simulink model "cx06_MA"  (Simulink 7.5)
settings: Solver=FixedStepDiscrete  StartTime=0.0  StopTime=10.0  RelTol=1e-3
undefined symbols (not defined in the file or in its folder): DiscIntNeverNeededParam, ECU555, int, motohawk_build_version, motohawk_trunc_name, motohawk_vardec_path
libraries: MotoHawk_lib x811, simulink x43, simulink_need_slupdate x1
(part 10 of 10)

== system cx06_MA/Strategy/Hybrid Control Code/Regen/SOC_RampOut ==
  Torque_In : Inport  OutDataType=sfix(16)  OutScaling=2^0
  SOC : Inport  Port=2  OutDataType=sfix(16)  OutScaling=2^0
  Constant : Constant  OutDataType=sfix(16)  OutScaling=2^0
  Divide : Product  Inputs=*/  OutDataType=sfix(16)  OutScaling=2^-10
  Product : Product  OutDataType=sfix(16)  OutScaling=2^0  RndMeth=Zero
  Relational Operator : RelationalOperator  Operator=<=  LogicOutDataTypeMode=boolean  OutDataTypeStr=boolean
  Saturation : Saturate  UpperLimit=1  LowerLimit=0
  Sum : Sum  Inputs=-++  OutDataType=sfix(16)  OutScaling=2^0
  Switch : Switch  Criteria=u2 ~= 0
  motohawk_calibration : MotoHawk_lib/Calibration & Probing Blocks/motohawk_calibration  nam='RegenSOCRampWidth'  val=5  storage=Calibration  show_more=on  name_source=Use Parameter  data_type=Inherit from 'Default Value'  read_level=1  write_level=1  ovr_cals=on  view_as=Number  enum_struct={'Disabled', 'Enabled'}  vector_style=Wide Row  use_help_units=on  help='Regen ramps out this fast over max SOC'  units='%'  use_header_enum=off  row_header_enum={}  col_header_enum={}  use_min_max=on  min_val=0  max_val=100  use_precision=off  precision=''  gain=1  offset=0  exp=1  use_mototune_group=off  mototune_group=motohawk_vardec_path(gcb)
  motohawk_calibration1 : MotoHawk_lib/Calibration & Probing Blocks/motohawk_calibration  nam='RegenMaxSOC'  val=90  storage=Calibration  show_more=on  name_source=Use Parameter  data_type=Inherit from 'Default Value'  read_level=1  write_level=1  ovr_cals=on  view_as=Number  enum_struct={'Disabled', 'Enabled'}  vector_style=Wide Row  use_help_units=on  help='Max SOC to Regen At'  units='%'  use_header_enum=off  row_header_enum={}  col_header_enum={}  use_min_max=on  min_val=0  max_val=100  use_precision=off  precision=''  gain=1  offset=0  exp=1  use_mototune_group=off  mototune_group=motohawk_vardec_path(gcb)
  Torque_Out : Outport  OutDataType=sfix(16)  OutScaling=2^0
  wires:
  Product/1 -> Torque_Out/1
  Switch/1 -> Saturation/1
  Torque_In/1 -> Product/1
  Constant/1 -> Switch/1
  Divide/1 -> Switch/3
  Relational Operator/1 -> Switch/2
  motohawk_calibration/1 -> Divide/2, Sum/3
  Sum/1 -> Divide/1
  SOC/1 -> Sum/1, Relational Operator/1
  motohawk_calibration1/1 -> Sum/2, Relational Operator/2
  Saturation/1 -> Product/2

== system cx06_MA/Strategy/Hybrid Control Code/Regen/speed_RampOut ==
  note: Include a sign reversal for reverse regen here.
      | This will keep a consistant pedal feel.
  Torque_In : Inport  OutDataType=sfix(16)  OutScaling=2^0
  speed : Inport  Port=2  OutDataType=sfix(16)  OutScaling=2^0
  Abs : Abs
  Constant : Constant  OutDataType=sfix(16)  OutScaling=2^0
  Divide : Product  Inputs=*/  OutDataType=sfix(16)  OutScaling=2^-10
  Product : Product  Inputs=3  OutDataType=sfix(16)  OutScaling=2^0  RndMeth=Zero
  Relational Operator : RelationalOperator  Operator=>  LogicOutDataTypeMode=boolean  OutDataTypeStr=boolean
  Saturation : Saturate  UpperLimit=1  LowerLimit=0
  Sign : Signum
  Sum : Sum  Inputs=+-  OutDataType=sfix(16)  OutScaling=2^0
  Sum1 : Sum  Inputs=-+  OutDataType=sfix(16)  OutScaling=2^0
  Switch : Switch  Criteria=u2 ~= 0
  motohawk_data_def : MotoHawk_lib/Data Storage Blocks/motohawk_data_def  nam='RegenSpdRampStop'  container_nam=''  data=2  typ=double  struct_nam='MyStruct'  storage=NonVolatile  outputRef=off  use_vardec=on  window=Calibration  read_level=1  write_level=1  ovr_cals=on  view_as=Number  enum_struct={'Disabled', 'Enabled'}  vector_style=Wide Row  use_help_units=on  help='Speed at which regen is ramped out'  units='mph'  use_header_enum=off  row_header_enum=''  col_header_enum=''  use_min_max=on  min_val=0  max_val=100  use_precision=on  precision=''  gain=1  offset=0  exp=1  use_mototune_group=off  mototune_group=motohawk_vardec_path(gcb)  eval_name=RegenSpdRampStop  data_stores=motohawk_sfun_data_def_data_stores  struct_instances=motohawk_sfun_data_def_struct_instances  vardecs=motohawk_sfun_data_def_vardecs
  motohawk_data_def1 : MotoHawk_lib/Data Storage Blocks/motohawk_data_def  nam='RegenSpdRampStart'  container_nam=''  data=5  typ=double  struct_nam='MyStruct'  storage=NonVolatile  outputRef=off  use_vardec=on  window=Calibration  read_level=1  write_level=1  ovr_cals=on  view_as=Number  enum_struct={'Disabled', 'Enabled'}  vector_style=Wide Row  use_help_units=on  help='Speed at which regen starts to ramp out'  units='mph'  use_header_enum=off  row_header_enum=''  col_header_enum=''  use_min_max=off  min_val=0  max_val=100  use_precision=off  precision=''  gain=1  offset=0  exp=1  use_mototune_group=off  mototune_group=motohawk_vardec_path(gcb)  eval_name=RegenSpdRampStart  data_stores=motohawk_sfun_data_def_data_stores  struct_instances=motohawk_sfun_data_def_struct_instances  vardecs=motohawk_sfun_data_def_vardecs
  motohawk_data_read : MotoHawk_lib/Data Storage Blocks/motohawk_data_read  source=Lookup By Name  structure=Scalar  operation=Read scalar from location by index  sz_vec=4  sz_row=2  sz_col=3  typ=double  nam='RegenSpdRampStop'  checkNull=on  struct_inst_name='Struct1'  struct_nam='MyStruct'
  motohawk_data_read1 : MotoHawk_lib/Data Storage Blocks/motohawk_data_read  source=Lookup By Name  structure=Scalar  operation=Read scalar from location by index  sz_vec=4  sz_row=2  sz_col=3  typ=double  nam='RegenSpdRampStart'  checkNull=on  struct_inst_name='Struct1'  struct_nam='MyStruct'
  Torque_Out : Outport  OutDataType=sfix(16)  OutScaling=2^0
  wires:
  speed/1 -> Abs/1, Sign/1
  motohawk_data_read/1 -> Sum/2, Sum1/1
  motohawk_data_read1/1 -> Sum1/2, Relational Operator/2
  Sum/1 -> Divide/1
  Sum1/1 -> Divide/2
  Relational Operator/1 -> Switch/2
  Divide/1 -> Switch/3
  Constant/1 -> Switch/1
  Abs/1 -> Sum/1, Relational Operator/1
  Torque_In/1 -> Product/1
  Sign/1 -> Product/2
  Switch/1 -> Saturation/1
  Product/1 -> Torque_Out/1
  Saturation/1 -> Product/3

== system cx06_MA/Strategy/Hybrid Control Code/Traction Control/Manual Torque Override ==
  note: 1 = Manual, simplified
      | 0 = Automatic, Complex
  F_In : Inport  OutDataType=sfix(16)  OutScaling=2^0
  R_In : Inport  Port=2  OutDataType=sfix(16)  OutScaling=2^0
  Switch : Switch  Criteria=u2 > Threshold
  Switch1 : Switch  Criteria=u2 > Threshold
  motohawk_calibration1 : MotoHawk_lib/Calibration & Probing Blocks/motohawk_calibration  nam='R_Torque_Allowed'  val=1  storage=Calibration  show_more=on  name_source=Use Parameter  data_type=double  read_level=1  write_level=1  ovr_cals=on  view_as=Number  enum_struct={'Complex', 'Simplified')  vector_style=Wide Row  use_help_units=on  help='Max Torque allowed for Fiat, decimal from 0.0 -> 1.0'  units=''  use_header_enum=on  row_header_enum={}  col_header_enum={}  use_min_max=on  min_val=0  max_val=1  use_precision=off  precision=''  gain=1  offset=0  exp=1  use_mototune_group=off  mototune_group=motohawk_vardec_path(gcb)
  motohawk_calibration5 : MotoHawk_lib/Calibration & Probing Blocks/motohawk_calibration  nam='F_Torque_Allowed'  val=1  storage=Calibration  show_more=on  name_source=Use Parameter  data_type=double  read_level=1  write_level=1  ovr_cals=on  view_as=Number  enum_struct={'Complex', 'Simplified')  vector_style=Wide Row  use_help_units=on  help='Max Torque allowed for Fiat, decimal from 0.0 -> 1.0'  units=''  use_header_enum=on  row_header_enum={}  col_header_enum={}  use_min_max=on  min_val=0  max_val=1  use_precision=off  precision=''  gain=1  offset=0  exp=1  use_mototune_group=off  mototune_group=motohawk_vardec_path(gcb)
  motohawk_data_read1 : MotoHawk_lib/Data Storage Blocks/motohawk_data_read  source=Lookup By Name  structure=Scalar  operation=Read scalar from location by index  sz_vec=4  sz_row=2  sz_col=3  typ=uint8  nam='TCVersion'  checkNull=on  struct_inst_name='Struct1'  struct_nam='MyStruct'
  F_Torque_Limit : Outport  OutDataType=sfix(16)  OutScaling=2^0
  R_Torque_Limit : Outport  Port=2  OutDataType=sfix(16)  OutScaling=2^0
  wires:
  Switch/1 -> F_Torque_Limit/1
  motohawk_data_read1/1 -> Switch/2, Switch1/2
  R_In/1 -> Switch1/3
  Switch1/1 -> R_Torque_Limit/1
  F_In/1 -> Switch/3
  motohawk_calibration5/1 -> Switch/1
  motohawk_calibration1/1 -> Switch1/1

== system cx06_MA/Strategy/Hybrid Control Code/ZEV/SOC_RampOut ==
  Torque_In : Inport  OutDataType=sfix(16)  OutScaling=2^0
  SOC : Inport  Port=2  OutDataType=sfix(16)  OutScaling=2^0
  Constant : Constant  OutDataType=sfix(16)  OutScaling=2^0
  Divide : Product  Inputs=*/  OutDataType=sfix(16)  OutScaling=2^-10
  Product : Product  OutDataType=sfix(16)  OutScaling=2^0  RndMeth=Zero
  Relational Operator : RelationalOperator  Operator=>  LogicOutDataTypeMode=boolean  OutDataTypeStr=boolean
  Saturation : Saturate  UpperLimit=1  LowerLimit=0
  Sum : Sum  Inputs=+-+  OutDataType=sfix(16)  OutScaling=2^0
  Switch : Switch  Criteria=u2 ~= 0
  motohawk_calibration : MotoHawk_lib/Calibration & Probing Blocks/motohawk_calibration  nam='ZEVSOCRampWidth'  val=5  storage=Calibration  show_more=on  name_source=Use Parameter  data_type=Inherit from 'Default Value'  read_level=1  write_level=1  ovr_cals=on  view_as=Number  enum_struct={'Disabled', 'Enabled'}  vector_style=Wide Row  use_help_units=on  help='Assist ramps out this fast below min'  units='%'  use_header_enum=off  row_header_enum={}  col_header_enum={}  use_min_max=on  min_val=0  max_val=100  use_precision=off  precision=''  gain=1  offset=0  exp=1  use_mototune_group=off  mototune_group=motohawk_vardec_path(gcb)
  motohawk_calibration1 : MotoHawk_lib/Calibration & Probing Blocks/motohawk_calibration  nam='ZEVMinSOC'  val=37  storage=Calibration  show_more=on  name_source=Use Parameter  data_type=Inherit from 'Default Value'  read_level=1  write_level=1  ovr_cals=on  view_as=Number  enum_struct={'Disabled', 'Enabled'}  vector_style=Wide Row  use_help_units=on  help='Minimum SOC to assist'  units='%'  use_header_enum=off  row_header_enum={}  col_header_enum={}  use_min_max=on  min_val=0  max_val=100  use_precision=off  precision=''  gain=1  offset=0  exp=1  use_mototune_group=off  mototune_group=motohawk_vardec_path(gcb)
  Torque_Out : Outport  OutDataType=sfix(16)  OutScaling=2^0
  wires:
  SOC/1 -> Sum/1, Relational Operator/1
  motohawk_calibration1/1 -> Sum/2, Relational Operator/2
  motohawk_calibration/1 -> Divide/2, Sum/3
  Sum/1 -> Divide/1
  Relational Operator/1 -> Switch/2
  Divide/1 -> Switch/3
  Constant/1 -> Switch/1
  Torque_In/1 -> Product/1
  Switch/1 -> Saturation/1
  Product/1 -> Torque_Out/1
  Saturation/1 -> Product/2

== system cx06_MA/Strategy/Hybrid Control Code/sustain Brake/speed_RampOut ==
  Torque_In : Inport  OutDataType=sfix(16)  OutScaling=2^0
  speed : Inport  Port=2  OutDataType=sfix(16)  OutScaling=2^0
  Abs : Abs
  Constant : Constant  OutDataType=sfix(16)  OutScaling=2^0
  Divide : Product  Inputs=*/  OutDataType=sfix(16)  OutScaling=2^-10
  Product : Product  Inputs=3  OutDataType=sfix(16)  OutScaling=2^0  RndMeth=Zero
  Relational Operator : RelationalOperator  Operator=>  LogicOutDataTypeMode=boolean  OutDataTypeStr=boolean
  Saturation : Saturate  UpperLimit=1  LowerLimit=0
  Sign : Signum
  Sum : Sum  Inputs=+-  OutDataType=sfix(16)  OutScaling=2^0
  Sum1 : Sum  Inputs=-+  OutDataType=sfix(16)  OutScaling=2^0
  Switch : Switch  Criteria=u2 > Threshold
  motohawk_data_read : MotoHawk_lib/Data Storage Blocks/motohawk_data_read  source=Lookup By Name  structure=Scalar  operation=Read scalar from location by index  sz_vec=4  sz_row=2  sz_col=3  typ=double  nam='RegenSpdRampStop'  checkNull=on  struct_inst_name='Struct1'  struct_nam='MyStruct'
  motohawk_data_read1 : MotoHawk_lib/Data Storage Blocks/motohawk_data_read  source=Lookup By Name  structure=Scalar  operation=Read scalar from location by index  sz_vec=4  sz_row=2  sz_col=3  typ=double  nam='RegenSpdRampStart'  checkNull=on  struct_inst_name='Struct1'  struct_nam='MyStruct'
  Torque_Out : Outport  OutDataType=sfix(16)  OutScaling=2^0
  wires:
  speed/1 -> Abs/1, Sign/1
  motohawk_data_read/1 -> Sum/2, Sum1/1
  motohawk_data_read1/1 -> Sum1/2, Relational Operator/2
  Sum/1 -> Divide/1
  Sum1/1 -> Divide/2
  Relational Operator/1 -> Switch/2
  Divide/1 -> Switch/3
  Constant/1 -> Switch/1
  Abs/1 -> Sum/1, Relational Operator/1
  Torque_In/1 -> Product/1
  Sign/1 -> Product/2
  Switch/1 -> Saturation/1
  Product/1 -> Torque_Out/1
  Saturation/1 -> Product/3

== system cx06_MA/Inputs/Analog Inputs/Driver Inputs/Accel/Range_Detect ==
  Value : Inport  OutDataType=sfix(16)  OutScaling=2^0
  Zero : Inport  Port=2  OutDataType=sfix(16)  OutScaling=2^0
  Full : Inport  Port=3  OutDataType=sfix(16)  OutScaling=2^0
  Gain : Gain  Gain=0.1  ParameterDataType=sfix(16)  ParameterScaling=2^0  OutDataType=sfix(16)  OutScaling=2^0
  Logical Operator : Logic  Operator=OR  AllPortsSameDT=off  OutDataTypeMode=boolean  OutDataTypeStr=boolean
  MinMax : MinMax  Inputs=2  OutDataType=sfix(16)  OutScaling=2^0
  MinMax1 : MinMax  Function=max  Inputs=2  OutDataType=sfix(16)  OutScaling=2^0
  Relational Operator : RelationalOperator  Operator=>  LogicOutDataTypeMode=boolean  OutDataTypeStr=boolean
  Relational Operator1 : RelationalOperator  Operator=>  LogicOutDataTypeMode=boolean  OutDataTypeStr=boolean
  Sum : Sum  Inputs=|+-  OutDataType=sfix(16)  OutScaling=2^0
  Sum1 : Sum  Inputs=-+  OutDataType=sfix(16)  OutScaling=2^0
  Sum2 : Sum  Inputs=++|  OutDataType=sfix(16)  OutScaling=2^0
  Fault : Outport  OutDataType=sfix(16)  OutScaling=2^0
  wires:
  Zero/1 -> MinMax/1, MinMax1/2
  Full/1 -> MinMax/2, MinMax1/1
  MinMax/1 -> Sum1/1, Sum/1
  MinMax1/1 -> Sum1/2, Sum2/2
  Sum1/1 -> Gain/1
  Gain/1 -> Sum/2, Sum2/1
  Sum2/1 -> Relational Operator1/2
  Sum/1 -> Relational Operator/1
  Value/1 -> Relational Operator/2, Relational Operator1/1
  Relational Operator/1 -> Logical Operator/1
  Relational Operator1/1 -> Logical Operator/2
  Logical Operator/1 -> Fault/1

== system cx06_MA/Inputs/Analog Inputs/Driver Inputs/Accel/Range_Detect1 ==
  Value : Inport  OutDataType=sfix(16)  OutScaling=2^0
  Zero : Inport  Port=2  OutDataType=sfix(16)  OutScaling=2^0
  Full : Inport  Port=3  OutDataType=sfix(16)  OutScaling=2^0
  Gain : Gain  Gain=0.1  ParameterDataType=sfix(16)  ParameterScaling=2^0  OutDataType=sfix(16)  OutScaling=2^0
  Logical Operator : Logic  Operator=OR  AllPortsSameDT=off  OutDataTypeMode=boolean  OutDataTypeStr=boolean
  MinMax : MinMax  Inputs=2  OutDataType=sfix(16)  OutScaling=2^0
  MinMax1 : MinMax  Function=max  Inputs=2  OutDataType=sfix(16)  OutScaling=2^0
  Relational Operator : RelationalOperator  Operator=>  LogicOutDataTypeMode=boolean  OutDataTypeStr=boolean
  Relational Operator1 : RelationalOperator  Operator=>  LogicOutDataTypeMode=boolean  OutDataTypeStr=boolean
  Sum : Sum  Inputs=|+-  OutDataType=sfix(16)  OutScaling=2^0
  Sum1 : Sum  Inputs=-+  OutDataType=sfix(16)  OutScaling=2^0
  Sum2 : Sum  Inputs=++|  OutDataType=sfix(16)  OutScaling=2^0
  Fault : Outport  OutDataType=sfix(16)  OutScaling=2^0
  wires:
  Logical Operator/1 -> Fault/1
  Relational Operator1/1 -> Logical Operator/2
  Relational Operator/1 -> Logical Operator/1
  Value/1 -> Relational Operator1/1, Relational Operator/2
  Sum/1 -> Relational Operator/1
  Sum2/1 -> Relational Operator1/2
  Gain/1 -> Sum2/1, Sum/2
  Sum1/1 -> Gain/1
  MinMax1/1 -> Sum2/2, Sum1/2
  MinMax/1 -> Sum/1, Sum1/1
  Full/1 -> MinMax1/1, MinMax/2
  Zero/1 -> MinMax1/2, MinMax/1

== system cx06_MA/Inputs/Analog Inputs/Driver Inputs/Brake/Range_Detect2 ==
  Value : Inport  OutDataType=sfix(16)  OutScaling=2^0
  Zero : Inport  Port=2  OutDataType=sfix(16)  OutScaling=2^0
  Full : Inport  Port=3  OutDataType=sfix(16)  OutScaling=2^0
  Gain : Gain  Gain=0.1  ParameterDataType=sfix(16)  ParameterScaling=2^0  OutDataType=sfix(16)  OutScaling=2^0
  Logical Operator : Logic  Operator=OR  AllPortsSameDT=off  OutDataTypeMode=boolean  OutDataTypeStr=boolean
  MinMax : MinMax  Inputs=2  OutDataType=sfix(16)  OutScaling=2^0
  MinMax1 : MinMax  Function=max  Inputs=2  OutDataType=sfix(16)  OutScaling=2^0
  Relational Operator : RelationalOperator  Operator=>  LogicOutDataTypeMode=boolean  OutDataTypeStr=boolean
  Relational Operator1 : RelationalOperator  Operator=>  LogicOutDataTypeMode=boolean  OutDataTypeStr=boolean
  Sum : Sum  Inputs=|+-  OutDataType=sfix(16)  OutScaling=2^0
  Sum1 : Sum  Inputs=-+  OutDataType=sfix(16)  OutScaling=2^0
  Sum2 : Sum  Inputs=++|  OutDataType=sfix(16)  OutScaling=2^0
  Fault : Outport  OutDataType=sfix(16)  OutScaling=2^0
  wires:
  Logical Operator/1 -> Fault/1
  Relational Operator1/1 -> Logical Operator/2
  Relational Operator/1 -> Logical Operator/1
  Value/1 -> Relational Operator1/1, Relational Operator/2
  Sum/1 -> Relational Operator/1
  Sum2/1 -> Relational Operator1/2
  Gain/1 -> Sum2/1, Sum/2
  Sum1/1 -> Gain/1
  MinMax1/1 -> Sum2/2, Sum1/2
  MinMax/1 -> Sum/1, Sum1/1
  Full/1 -> MinMax1/1, MinMax/2
  Zero/1 -> MinMax1/2, MinMax/1

== system cx06_MA/Inputs/Analog Inputs/Driver Inputs/Brake/Range_Detect5 ==
  Value : Inport  OutDataType=sfix(16)  OutScaling=2^0
  Zero : Inport  Port=2  OutDataType=sfix(16)  OutScaling=2^0
  Full : Inport  Port=3  OutDataType=sfix(16)  OutScaling=2^0
  Gain : Gain  Gain=0.1  ParameterDataType=sfix(16)  ParameterScaling=2^0  OutDataType=sfix(16)  OutScaling=2^0
  Logical Operator : Logic  Operator=OR  AllPortsSameDT=off  OutDataTypeMode=boolean  OutDataTypeStr=boolean
  MinMax : MinMax  Inputs=2  OutDataType=sfix(16)  OutScaling=2^0
  MinMax1 : MinMax  Function=max  Inputs=2  OutDataType=sfix(16)  OutScaling=2^0
  Relational Operator : RelationalOperator  Operator=>  LogicOutDataTypeMode=boolean  OutDataTypeStr=boolean
  Relational Operator1 : RelationalOperator  Operator=>  LogicOutDataTypeMode=boolean  OutDataTypeStr=boolean
  Sum : Sum  Inputs=|+-  OutDataType=sfix(16)  OutScaling=2^0
  Sum1 : Sum  Inputs=-+  OutDataType=sfix(16)  OutScaling=2^0
  Sum2 : Sum  Inputs=++|  OutDataType=sfix(16)  OutScaling=2^0
  Fault : Outport  OutDataType=sfix(16)  OutScaling=2^0
  wires:
  Zero/1 -> MinMax/1, MinMax1/2
  Full/1 -> MinMax/2, MinMax1/1
  MinMax/1 -> Sum1/1, Sum/1
  MinMax1/1 -> Sum1/2, Sum2/2
  Sum1/1 -> Gain/1
  Gain/1 -> Sum/2, Sum2/1
  Sum2/1 -> Relational Operator1/2
  Sum/1 -> Relational Operator/1
  Value/1 -> Relational Operator/2, Relational Operator1/1
  Relational Operator/1 -> Logical Operator/1
  Relational Operator1/1 -> Logical Operator/2
  Logical Operator/1 -> Fault/1

== system cx06_MA/Inputs/Analog Inputs/Driver Inputs/Brake/Redundant_Check ==
  In1 : Inport  OutDataType=sfix(16)  OutScaling=2^0
  Allowable_Error : Inport  Port=2  OutDataType=sfix(16)  OutScaling=2^0
  In2 : Inport  Port=3  OutDataType=sfix(16)  OutScaling=2^0
  Abs : Abs
  Relational Operator : RelationalOperator  Operator=>  LogicOutDataTypeMode=boolean  OutDataTypeStr=boolean
  Sum1 : Sum  Inputs=+-  OutDataType=sfix(16)  OutScaling=2^0
  Fault : Outport  OutDataType=sfix(16)  OutScaling=2^0
  wires:
  In2/1 -> Sum1/2
  In1/1 -> Sum1/1
  Sum1/1 -> Abs/1
  Allowable_Error/1 -> Relational Operator/2
  Abs/1 -> Relational Operator/1
  Relational Operator/1 -> Fault/1

== system cx06_MA/Inputs/Analog Inputs/Driver Inputs/Clutch/Range_Detect3 ==
  Value : Inport  OutDataType=sfix(16)  OutScaling=2^0
  Zero : Inport  Port=2  OutDataType=sfix(16)  OutScaling=2^0
  Full : Inport  Port=3  OutDataType=sfix(16)  OutScaling=2^0
  Gain : Gain  Gain=0.1  ParameterDataType=sfix(16)  ParameterScaling=2^0  OutDataType=sfix(16)  OutScaling=2^0
  Logical Operator : Logic  Operator=OR  AllPortsSameDT=off  OutDataTypeMode=boolean  OutDataTypeStr=boolean
  MinMax : MinMax  Inputs=2  OutDataType=sfix(16)  OutScaling=2^0
  MinMax1 : MinMax  Function=max  Inputs=2  OutDataType=sfix(16)  OutScaling=2^0
  Relational Operator : RelationalOperator  Operator=>  LogicOutDataTypeMode=boolean  OutDataTypeStr=boolean
  Relational Operator1 : RelationalOperator  Operator=>  LogicOutDataTypeMode=boolean  OutDataTypeStr=boolean
  Sum : Sum  Inputs=|+-  OutDataType=sfix(16)  OutScaling=2^0
  Sum1 : Sum  Inputs=-+  OutDataType=sfix(16)  OutScaling=2^0
  Sum2 : Sum  Inputs=++|  OutDataType=sfix(16)  OutScaling=2^0
  Fault : Outport  OutDataType=sfix(16)  OutScaling=2^0
  wires:
  Zero/1 -> MinMax/1, MinMax1/2
  Full/1 -> MinMax/2, MinMax1/1
  MinMax/1 -> Sum1/1, Sum/1
  MinMax1/1 -> Sum1/2, Sum2/2
  Sum1/1 -> Gain/1
  Gain/1 -> Sum/2, Sum2/1
  Sum2/1 -> Relational Operator1/2
  Sum/1 -> Relational Operator/1
  Value/1 -> Relational Operator/2, Relational Operator1/1
  Relational Operator/1 -> Logical Operator/1
  Relational Operator1/1 -> Logical Operator/2
  Logical Operator/1 -> Fault/1

== system cx06_MA/Inputs/Analog Inputs/Driver Inputs/Clutch/Range_Detect4 ==
  Value : Inport  OutDataType=sfix(16)  OutScaling=2^0
  Zero : Inport  Port=2  OutDataType=sfix(16)  OutScaling=2^0
  Full : Inport  Port=3  OutDataType=sfix(16)  OutScaling=2^0
  Gain : Gain  Gain=0.1  ParameterDataType=sfix(16)  ParameterScaling=2^0  OutDataType=sfix(16)  OutScaling=2^0
  Logical Operator : Logic  Operator=OR  AllPortsSameDT=off  OutDataTypeMode=boolean  OutDataTypeStr=boolean
  MinMax : MinMax  Inputs=2  OutDataType=sfix(16)  OutScaling=2^0
  MinMax1 : MinMax  Function=max  Inputs=2  OutDataType=sfix(16)  OutScaling=2^0
  Relational Operator : RelationalOperator  Operator=>  LogicOutDataTypeMode=boolean  OutDataTypeStr=boolean
  Relational Operator1 : RelationalOperator  Operator=>  LogicOutDataTypeMode=boolean  OutDataTypeStr=boolean
  Sum : Sum  Inputs=|+-  OutDataType=sfix(16)  OutScaling=2^0
  Sum1 : Sum  Inputs=-+  OutDataType=sfix(16)  OutScaling=2^0
  Sum2 : Sum  Inputs=++|  OutDataType=sfix(16)  OutScaling=2^0
  Fault : Outport  OutDataType=sfix(16)  OutScaling=2^0
  wires:
  Zero/1 -> MinMax/1, MinMax1/2
  Full/1 -> MinMax/2, MinMax1/1
  MinMax/1 -> Sum1/1, Sum/1
  MinMax1/1 -> Sum1/2, Sum2/2
  Sum1/1 -> Gain/1
  Gain/1 -> Sum/2, Sum2/1
  Sum2/1 -> Relational Operator1/2
  Sum/1 -> Relational Operator/1
  Value/1 -> Relational Operator/2, Relational Operator1/1
  Relational Operator/1 -> Logical Operator/1
  Relational Operator1/1 -> Logical Operator/2
  Logical Operator/1 -> Fault/1

== system cx06_MA/Inputs/Analog Inputs/Driver Inputs/Clutch/Redundant_Check ==
  In1 : Inport  OutDataType=sfix(16)  OutScaling=2^0
  Allowable_Error : Inport  Port=2  OutDataType=sfix(16)  OutScaling=2^0
  In2 : Inport  Port=3  OutDataType=sfix(16)  OutScaling=2^0
  Abs : Abs
  Relational Operator : RelationalOperator  Operator=>  LogicOutDataTypeMode=boolean  OutDataTypeStr=boolean
  Sum1 : Sum  Inputs=+-  OutDataType=sfix(16)  OutScaling=2^0
  Fault : Outport  OutDataType=sfix(16)  OutScaling=2^0
  wires:
  In2/1 -> Sum1/2
  In1/1 -> Sum1/1
  Sum1/1 -> Abs/1
  Allowable_Error/1 -> Relational Operator/2
  Abs/1 -> Relational Operator/1
  Relational Operator/1 -> Fault/1

== system cx06_MA/Strategy/Hybrid Control Code/Activation of Traction Control/Wheel_Acceleration/motorTorqueFilter ==
  In1 : Inport  OutDataType=sfix(16)  OutScaling=2^0
  K_Value : Inport  Port=2  OutDataType=sfix(16)  OutScaling=2^0
  Constant : Constant  OutDataType=sfix(16)  OutScaling=2^0
  Product : Product  OutDataType=sfix(16)  OutScaling=2^0  RndMeth=Zero
  Product1 : Product  OutDataType=sfix(16)  OutScaling=2^0  RndMeth=Zero
  Sum : Sum  Inputs=|++  OutDataType=sfix(16)  OutScaling=2^0
  Sum1 : Sum  Inputs=|-+  OutDataType=sfix(16)  OutScaling=2^0
  Unit Delay1 : UnitDelay  SampleTime=-1
  Out1 : Outport  OutDataType=sfix(16)  OutScaling=2^0
  wires:
  In1/1 -> Product/1
  K_Value/1 -> Product/2, Sum1/1
  Product/1 -> Sum/1
  Constant/1 -> Sum1/2
  Sum1/1 -> Product1/1
  Product1/1 -> Sum/2
  Unit Delay1/1 -> Product1/2
  Sum/1 -> Unit Delay1/1, Out1/1

== system cx06_MA/Strategy/Hybrid Control Code/Activation of Traction Control/Wheel_Acceleration/motorTorqueFilter1 ==
  In1 : Inport  OutDataType=sfix(16)  OutScaling=2^0
  K_Value : Inport  Port=2  OutDataType=sfix(16)  OutScaling=2^0
  Constant : Constant  OutDataType=sfix(16)  OutScaling=2^0
  Product : Product  OutDataType=sfix(16)  OutScaling=2^0  RndMeth=Zero
  Product1 : Product  OutDataType=sfix(16)  OutScaling=2^0  RndMeth=Zero
  Sum : Sum  Inputs=|++  OutDataType=sfix(16)  OutScaling=2^0
  Sum1 : Sum  Inputs=|-+  OutDataType=sfix(16)  OutScaling=2^0
  Unit Delay1 : UnitDelay  SampleTime=-1
  Out1 : Outport  OutDataType=sfix(16)  OutScaling=2^0
  wires:
  In1/1 -> Product/1
  K_Value/1 -> Product/2, Sum1/1
  Product/1 -> Sum/1
  Constant/1 -> Sum1/2
  Sum1/1 -> Product1/1
  Product1/1 -> Sum/2
  Unit Delay1/1 -> Product1/2
  Sum/1 -> Unit Delay1/1, Out1/1

== system cx06_MA/Strategy/Hybrid Control Code/Activation of Traction Control/Wheel_Acceleration/motorTorqueFilter2 ==
  In1 : Inport  OutDataType=sfix(16)  OutScaling=2^0
  K_Value : Inport  Port=2  OutDataType=sfix(16)  OutScaling=2^0
  Constant : Constant  OutDataType=sfix(16)  OutScaling=2^0
  Product : Product  OutDataType=sfix(16)  OutScaling=2^0  RndMeth=Zero
  Product1 : Product  OutDataType=sfix(16)  OutScaling=2^0  RndMeth=Zero
  Sum : Sum  Inputs=|++  OutDataType=sfix(16)  OutScaling=2^0
  Sum1 : Sum  Inputs=|-+  OutDataType=sfix(16)  OutScaling=2^0
  Unit Delay1 : UnitDelay  SampleTime=-1
  Out1 : Outport  OutDataType=sfix(16)  OutScaling=2^0
  wires:
  In1/1 -> Product/1
  K_Value/1 -> Product/2, Sum1/1
  Product/1 -> Sum/1
  Constant/1 -> Sum1/2
  Sum1/1 -> Product1/1
  Product1/1 -> Sum/2
  Unit Delay1/1 -> Product1/2
  Sum/1 -> Unit Delay1/1, Out1/1

== system cx06_MA/Strategy/Hybrid Control Code/Activation of Traction Control/Wheel_Acceleration/motorTorqueFilter3 ==
  In1 : Inport  OutDataType=sfix(16)  OutScaling=2^0
  K_Value : Inport  Port=2  OutDataType=sfix(16)  OutScaling=2^0
  Constant : Constant  OutDataType=sfix(16)  OutScaling=2^0
  Product : Product  OutDataType=sfix(16)  OutScaling=2^0  RndMeth=Zero
  Product1 : Product  OutDataType=sfix(16)  OutScaling=2^0  RndMeth=Zero
  Sum : Sum  Inputs=|++  OutDataType=sfix(16)  OutScaling=2^0
  Sum1 : Sum  Inputs=|-+  OutDataType=sfix(16)  OutScaling=2^0
  Unit Delay1 : UnitDelay  SampleTime=-1
  Out1 : Outport  OutDataType=sfix(16)  OutScaling=2^0
  wires:
  In1/1 -> Product/1
  K_Value/1 -> Product/2, Sum1/1
  Product/1 -> Sum/1
  Constant/1 -> Sum1/2
  Sum1/1 -> Product1/1
  Product1/1 -> Sum/2
  Unit Delay1/1 -> Product1/2
  Sum/1 -> Unit Delay1/1, Out1/1

== stateflow chart MainState/Chart ==
  state PowerUp
    during:MS_State = 0;
    during:MPRD = 0;
  state On
    during:MS_State = 1;
    during:MPRD = 1;
  state Estop
    during:MS_State = 2
    during:MPRD = 0;
  state PowerDown
    during:MS_State = 3;
    during:MPRD = EStop;
  state ShutDown
    entry:Shutdown = 0;
    during:MPRD = 0;
  (default) -> PowerUp : {PowerUp}
  PowerUp -> On [order 1] : [EStop == 0]
  PowerUp -> Estop [order 2] : [EStop == 1]
  On -> Estop [order 2] : [EStop == 1]
  Estop -> On [order 1] : [EStop == 0]
  On -> PowerDown [order 1] : [Ecup == 0]
  Estop -> PowerDown [order 2] : [Ecup == 0]
  PowerDown -> ShutDown [order 2] : [PowerDown_Cmplt == 1]
  PowerDown -> Estop [order 3] : [(Ecup == 1)&...
      | (EStop == 1)]
  PowerDown -> On [order 1] : [(Ecup == 1)&...
      | (EStop == 0)]
  data: EStop input double; Ecup input double; MS_State output uint8; PowerDown_Cmplt input double; MPRD output boolean; Shutdown output boolean =1
  events: PowerUp output EITHER_EDGE_EVENT; PowerDown output EITHER_EDGE_EVENT

== stateflow chart Strategy/Hybrid Control Code/sustain Brake/Sustain Brake original ==
  state Off
    entry:SB = 0;
    during:level = max(level-1/(ramp_time), 0);
  state On
    entry:SB = 1;
    during:level = min(level+1/(ramp_time), 1);
  Off -> On : [SOC < SB_On]
  On -> Off : [SOC > SB_Off]
  (default) -> Off
  data: SOC input double; SB_Off input double; SB_On input double; level output double; ramp_time input double; SB output uint8

== matlab function Strategy/Hybrid Control Code/hybrid State calc ==
  data: sport_mode input double; neutral input double; state output double; reverse input double; braking input double; clutching input double
function state = fcn(sport_mode, neutral, reverse, braking, clutching)
% This block supports an embeddable subset of the MATLAB language.
% See the help menu for details. 

%reverse assist possible implementation
%if(braking == 1)
%    state = 2;%regen
%elseif((neutral == 1) && (clutching == 0))
%    state = 4;%ZEV
%elseif((clutching == 1) && (sport_mode == 0))
%    state = 1;%diesel
%else
%    state = 3;%HEV
%end

%note: don't care about reverse (reverse is effectively any other gear)





%sport mode (5/22/2007)
if(braking == 1)
    state = 2;%regen
elseif (reverse == 1)
    state = 1;%diesel
elseif((neutral == 1) && (clutching == 0))
    state = 4;%ZEV
elseif((clutching == 1) && (sport_mode == 0))
    state = 1;%diesel
else
    state = 3;%HEV
end

== matlab function Outputs/GMLAN Outputs/Act_Gear_Translate ==
  data: u input double; y output double
function y = fcn(u)
% This block supports an embeddable subset of the MATLAB language.
% See the help menu for details. 

if(u == -1)
    y = 8;
elseif(u == 0)
    y = 9;
elseif(u <=6)
    y = double(u);
else
    y = 0;
end

== matlab function Outputs/GMLAN Outputs/Cmd_Gear_Translate ==
  data: u input double; y output double
function y = fcn(u)
% This block supports an embeddable subset of the MATLAB language.
% See the help menu for details. 

if((u > 0) && (u <=6))
    y = double(u);
else
    y = 0;
end

== matlab function Outputs/GMLAN Outputs/Gear_Pos_Translate ==
  data: u input double; y output double
function y = fcn(u)
% This block supports an embeddable subset of the MATLAB language.
% See the help menu for details. 

if(u == -1)
    y = 8;
elseif(u == 0)
    y = 9;
elseif(u <=6)
    y = double(u);
else
    y = 0;
end

== matlab function Strategy/Hybrid Control Code/HEV/AssistedTakeOff/Embedded MATLAB Function ==
  data: clutch input double; sw output double; start input double; full input double; ramp input double; stop input double
function sw = fcn(clutch, start, full, ramp, stop)
% This block supports an embeddable subset of the MATLAB language.
% See the help menu for details. 

if(clutch > start)
    sw = 1;
elseif(clutch > full)
    sw = 2;
elseif(clutch > ramp)
    sw = 3;
elseif(clutch > stop)
    sw = 4;
else
    sw = 5;
end

== stateflow chart Strategy/Hybrid Control Code/Activation of Assisted Take-off/Chart ==
  state Off
    entry:active = 0;
  state On
    entry:active = 1;
  (default) -> Off
  On -> Off : [clutch < Stop]
  Off -> On : [(clutch > Start)&...
      | (speed < 2)&...
      | (enabled == 1)]
  data: Start input double; Stop input double; active output uint8; clutch input double; speed input double; enabled input double

== matlab function Strategy/Hybrid Control Code/Hybrid state limits/Embedded MATLAB Function ==
  data: state input double; nState output double; nDiesel input double; nHEV input double; nZEV input double; nRegen input double
function nState = fcn(state, nDiesel,nHEV,nZEV,nRegen)
% This block supports an embeddable subset of the MATLAB language.
% See the help menu for details. 

nState = state;
if((state == 2) && (nRegen == 1))
    nState = 1;
end
if((state == 3) && (nHEV == 1))
    nState = 1;
end
if((state == 4) && (nZEV == 1))
    nState = 1;
end
if((state == 1) && (nDiesel == 1))
    nState = 0;
end

== stateflow chart Strategy/Urea Control Code/LeanRich/Chart ==
  state Neutral
    entry:Ammonia = -1;
    entry:mult = 1;
    entry:State = 1;
  state Lean
    entry:Ammonia = 1;
    entry:mult = LeanMult;
    entry:State = 2;
  state Lean2Rich
    entry:Ammonia = 0;
    entry:LeanCnt = 0;
    entry:State = 3;
    during:LeanCnt = LeanCnt + 1;
  state Rich2Lean
    entry:Ammonia = 1;
    entry:RichCnt = 0;
    entry:State = 4;
    during: RichCnt = RichCnt + 1;
  state Rich
    entry:Ammonia = 0;
    entry:State = 5;
    entry:mult = RichMult;
  state Error
    entry:Ammonia = -1;
    entry:mult = 1;
    entry:State = 6;
  (default) -> Neutral
  Neutral -> Lean [order 1] : [(temp > minTemp)&...
      |  (NOx > NOxThres)]
  Lean -> Lean2Rich [order 2] : [NOx < NOxThres]
  Lean -> Neutral [order 3] : [temp < minTemp]
  Lean2Rich -> Lean [order 1] : [NOx > NOxThres]
  Neutral -> Rich [order 3] : [(temp > minTemp)&...
      |  (NOx < NOxThres)]
  Rich -> Neutral [order 1] : [temp < minTemp]
  Rich -> Rich2Lean [order 2] : [NOx > NOxThres]
  Rich2Lean -> Rich [order 3] : [NOx < NOxThres]
  Rich2Lean -> Lean2Rich [order 1] : [RichCnt > RichTime]
  Lean2Rich -> Rich2Lean [order 3] : [LeanCnt > LeanTime]
  Lean2Rich -> Neutral [order 4] : [temp < minTemp]
  Rich2Lean -> Neutral [order 4] : [temp < minTemp]
  Lean -> Error [order 1] : [errorIn == 1]
  Lean2Rich -> Error [order 2] : [errorIn == 1]
  Rich2Lean -> Error [order 2] : [errorIn == 1]
  Rich -> Error [order 3] : [errorIn == 1]
  Neutral -> Error [order 2] : [errorIn == 1]
  Error -> Neutral : [errorIn == 0]
  data: errorIn input boolean; NOx input double; temp input double; Ammonia output uint8; LeanCnt output uint16; LeanMult input double; LeanTime input double; RichCnt output uint16; RichMult input double; RichTime input double; NOxThres input double; minTemp input double; mult output double; State output uint8

== matlab function Inputs/Analog Inputs/Cruise Buttons/read_Cruise_Buttons ==
  data: u input double; cruiseBut output double; b1 input double; b2 input double; b3 input double
function cruiseBut = fcn(u, b1, b2, b3)
% This block supports an embeddable subset of the MATLAB language.
% See the help menu for details. 
cruiseBut = 0;
if(u > b1)
    cruiseBut = cruiseBut+1;
end
if(u > b2)
    cruiseBut = cruiseBut+1;
end
if(u > b3)
    cruiseBut = cruiseBut+1;
end

== stateflow chart Strategy/A/C Control Code/A/C StateMachine ==
  state Off
    entry:activate = 0;
  state On
    entry:activate = 1;
  Off -> On : [Pressure < on_Pres]
  On -> Off : [Pressure > off_Pres]
  (default) -> Off
  data: Pressure input double; off_Pres input double; on_Pres input double; activate output boolean

== stateflow chart Outputs/Analog Outputs/Backup_Relay_Control/Chart ==
  state Idle
    during: LSD_Eng= 0
    during: LSD_Nav = 1
    during: timer = 0
    during: state = 0
  state About_to_Idle
    during: LSD_Eng = 0
    during: LSD_Nav = 0
    during: timer = 1
    during: state = 3
  state About_to_Crank
    during: LSD_Eng = 0
    during: LSD_Nav = 0
    during: timer = 1
    during: state = 1
  state Crank
    during: LSD_Eng = 1
    during: LSD_Nav = 0
    during: timer = 0
    during: state = 2
  About_to_Idle -> Idle [order 1] : [Delay_2==1]
  Idle -> About_to_Crank : [Eng_Start == 1]
  About_to_Crank -> Crank [order 1] : [Delay_1 == 1]
  Crank -> About_to_Idle : [Eng_Start == 0]
  About_to_Idle -> Crank [order 2] : [Eng_Start == 1]
  About_to_Crank -> Idle [order 2] : [Eng_Start == 0]
  (default) -> Idle
  data: Eng_Start input double; Delay_1 input double; Delay_2 input double; LSD_Eng output uint8; LSD_Nav output uint8; timer output uint8; state output uint8

== stateflow chart Strategy/Hybrid Control Code/Engine Start-Stop/Engine_Running ==
  state NotRunning
    entry:running = 0;
  state Running
    entry:running = 1;
  (default) -> NotRunning
  Running -> NotRunning : [RPM < Stop_RPM]
  NotRunning -> Running : [RPM > Start_RPM]
  data: RPM input double; Start_RPM input double; Stop_RPM input double; running output uint8

== stateflow chart Strategy/Hybrid Control Code/Engine Start-Stop/Old_Alg/EngineSS_StateMachine ==
  state Idle
    entry:StartRetry_Cnt = StartRetry_Cnt...
    *(neutral == 1);
    during: ESS_State=0;
  state KillDelay
    entry:KillDelay_Cnt = 0;
    entry:StartRetry_Cnt = 0;
    during:KillDelay_Cnt++;
    during: ESS_State=4;
  state Kill
    entry:kill = 1;
    entry:Kill_Cnt = 0;
    during:Kill_Cnt++;
    exit:kill = 0;
    during: ESS_State=5;
  state StartDelay
    entry:StartDelay_Cnt = 0;
    during:StartDelay_Cnt++;
    during: ESS_State=1;
  state Start
    entry:start = 1;
    entry:Start_Cnt = 0;
    during:Start_Cnt++;
    exit:start= 0;
    during: ESS_State=2;
  state StartRetry
    entry:StartRetry_Cnt++;
    entry:StartRetryDelay_Cnt = 0;
    during:StartRetryDelay_Cnt++;
    during: ESS_State=3;
  Idle -> KillDelay [order 2] : [(running == 1)&...
      | (neutral == 1)]
  (default) -> Idle
  KillDelay -> Kill [order 2] : [KillDelay_Cnt > KillDelay]
  KillDelay -> Idle [order 1] : [(running == 0)|...
      | (neutral == 0)]
  Kill -> Idle : [Kill_Cnt > Kill_Time]
  Idle -> StartDelay [order 1] : [(running == 0)&...
      | (neutral == 0)&...
      | (clutching == 1)]
  StartDelay -> Idle [order 1] : [(running == 1)|...
      | (neutral == 1)|...
      | (clutching == 0)]
  StartDelay -> Start [order 2] : [StartDelay_Cnt > Start_Delay]
  Start -> StartRetry [order 2] : [Start_Cnt > Start_Time]
  StartRetry -> Idle : [((StartRetryDelay_Cnt > StartRetry_Delay)&...
      | (StartRetry_Cnt < Max_RetryCnt))|...
      | (neutral == 1)]
  Start -> Idle [order 1] : [running == 1]
  data: clutching input double; KillDelay input double; KillDelay_Cnt output double; Kill_Cnt output double; Kill_Time input double; Max_RetryCnt input double; StartDelay_Cnt output double; StartRetryDelay_Cnt output double; StartRetry_Cnt output double; StartRetry_Delay input double; Start_Cnt output double; Start_Delay input double; Start_Time input double; kill output double; neutral input double; running input double; start output double; ESS_State output uint8

== stateflow chart Outputs/IPT CAN Output/Disable_DCDC ==
  state Passthrough
    entry: cmd=0;
    during: cmd = 0;
  state Active
    entry: cmd=1;
    during: cmd=1;
  (default) -> Passthrough
  Passthrough -> Active : [SOC > On_SOC]
  Active -> Passthrough : [SOC < Off_SOC]
  data: SOC input double; On_SOC input double; Off_SOC input double; cmd output uint8

== stateflow chart Strategy/Hybrid Control Code/Engine Start-Stop/New_Alg/EngineSS_StateMachine1 ==
  state Idle
    entry:StartRetry_Cnt = StartRetry_Cnt...
    *(neutral == 1);
    during: ESS_State=0;
  state KillDelay
    entry:KillDelay_Cnt = 0;
    entry:StartRetry_Cnt = 0;
    during:KillDelay_Cnt++;
    during: ESS_State=4;
  state Kill
    entry:kill = 1;
    entry:Kill_Cnt = 0;
    during:Kill_Cnt++;
    exit:kill = 0;
    during: ESS_State=5;
  state StartDelay
    entry:StartDelay_Cnt = 0;
    during:StartDelay_Cnt++;
    during: ESS_State=1;
  state Start
    entry:start = 1;
    entry:Start_Cnt = 0;
    during:Start_Cnt++;
    exit:start= 0;
    during: ESS_State=2;
  state StartRetry
    entry:StartRetry_Cnt++;
    entry:StartRetryDelay_Cnt = 0;
    during:StartRetryDelay_Cnt++;
    during: ESS_State=3;
  state FalseStart
    during: ESS_State=6;
  Idle -> KillDelay [order 2] : [(running == 1)&...
      | (neutral == 1)&...
      | (clutching == 0)]
  (default) -> Idle
  KillDelay -> Kill [order 2] : [KillDelay_Cnt > KillDelay]
  KillDelay -> Idle [order 1] : [(running == 0)|...
      | (neutral == 0)]
  Kill -> Idle : [Kill_Cnt > Kill_Time]
  Idle -> StartDelay [order 1] : [(running == 0)&...
      | (clutching == 1)]
  StartDelay -> Idle [order 1] : [(running == 1)|...
      | (clutching == 0)]
  StartDelay -> Start [order 2] : [StartDelay_Cnt > Start_Delay]
  Start -> StartRetry [order 1] : [Start_Cnt > Start_Time]
  StartRetry -> Idle : [((StartRetryDelay_Cnt > StartRetry_Delay)&...
      | (StartRetry_Cnt < Max_RetryCnt))|...
      | (neutral == 1)]
  Start -> FalseStart [order 2] : [running == 1]
  FalseStart -> Idle : [(neutral == 0)|...
      | (running == 0)]
  data: clutching input double; KillDelay input double; KillDelay_Cnt output double; Kill_Cnt output double; Kill_Time input double; Max_RetryCnt input double; StartDelay_Cnt output double; StartRetryDelay_Cnt output double; StartRetry_Cnt output double; StartRetry_Delay input double; Start_Cnt output double; Start_Delay input double; Start_Time input double; kill output double; neutral input double; running input double; start output double; ESS_State output uint8

== stateflow chart Strategy/Hybrid Control Code/Activation of Accel Through Shifts/Engine_Running ==
  state OFF
    entry:output = spd;
    during: output = spd;
  state ON
    entry:output = 1;
    during: output = 1;
  (default) -> OFF
  ON -> OFF : [Braking | !Acceling]
  OFF -> ON : [Clutching & EBrake & !Braking & Acceling & !Neutral]
  data: output output uint8; Clutching input double; EBrake input double; Braking input double; Acceling input double; Neutral input double; spd input double

== matlab function Inputs/JCI CAN Input/SOC ==
  data: voltage input double; SOC output double; currentPlusMinus input double; lowV input double; highV input double; currentBat input double; SOCLast input double
function SOC  = fcn(voltage,currentPlusMinus,lowV,highV,currentBat,SOCLast)

if (currentBat<=currentPlusMinus && currentBat>=(-1*currentPlusMinus))
    SOC=(100*((voltage-lowV)/(highV-lowV)));
elseif (voltage>=390)
    SOC=100;
else
    SOC = SOCLast;
end
